simulink model "s1a"  (Simulink 2.00)
settings: Solver=ode15s  StartTime=0.0  StopTime=tstop  MaxStep=1e-3  RelTol=1e-8  AbsTol=1e-6
values from neighbouring files (symbols this model uses):
  Psi1o = 0    [M1.M]    (also in M4.M)
  Psip2o = 0    [M1.M]    (also in M4.M)
  r1 = 0.25    [M1.M]    (also in M4.M)
  rp2 = 0.134    [M1.M]    (also in M4.M)
  wb = 2*pi*Frated    (= 376.991118431)    [M1.M]    (also in M4.M)
  xl1 = 0.056    [M1.M]    (also in M4.M)
  xM = 1/(1/xm + 1/xl1 + 1/xpl2)    (= 0.0279988939489)    [M1.M]    (also in M4.M)
  xpl2 = 0.056    [M1.M]    (also in M4.M)
settings Model: SaveTime=off  SaveOutput=off  ConsistencyChecking=off

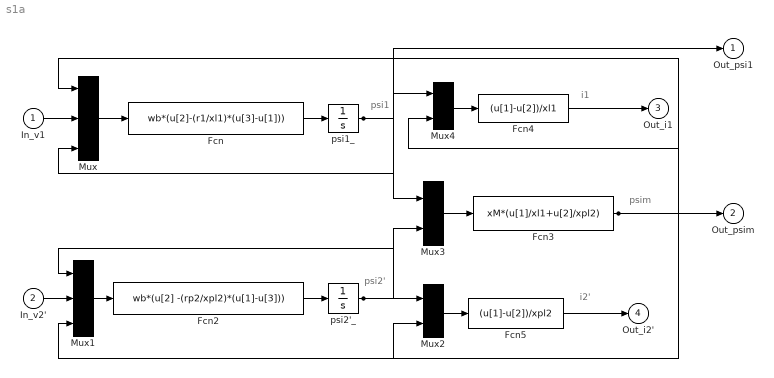
== system s1a ==
  note: i2'
  note: psi1
  note: psi2'
  note: i1
  note: psim
  In_v1 : Inport  Port=1  PortWidth=-1  SampleTime=-1
  In_v2' : Inport  Port=2  PortWidth=-1  SampleTime=-1
  Fcn : Fcn  Expr=wb*(u[2]-(r1/xl1)*(u[3]-u[1]))
  Fcn2 : Fcn  Expr=wb*(u[2] -(rp2/xpl2)*(u[1]-u[3]))
  Fcn3 : Fcn  Expr=xM*(u[1]/xl1+u[2]/xpl2)
  Fcn4 : Fcn  Expr=(u[1]-u[2])/xl1
  Fcn5 : Fcn  Expr=(u[1]-u[2])/xpl2
  Mux : Mux  Inputs=3
  Mux1 : Mux  Inputs=3
  Mux2 : Mux  Inputs=2
  Mux3 : Mux  Inputs=2
  Mux4 : Mux  Inputs=2
  psi1_ : Integrator  ExternalReset=none  InitialConditionSource=internal  InitialCondition=Psi1o  LimitOutput=off  UpperSaturationLimit=inf  LowerSaturationLimit=-inf  ShowSaturationPort=off  ShowStatePort=off  AbsoluteTolerance=auto
  psi2'_ : Integrator  ExternalReset=none  InitialConditionSource=internal  InitialCondition=Psip2o  LimitOutput=off  UpperSaturationLimit=inf  LowerSaturationLimit=-inf  ShowSaturationPort=off  ShowStatePort=off  AbsoluteTolerance=auto
  Out_psi1 : Outport  Port=1  InitialOutput=0
  Out_psim : Outport  Port=2  InitialOutput=0
  Out_i1 : Outport  Port=3  InitialOutput=0
  Out_i2' : Outport  Port=4  InitialOutput=0
  wires:
  In_v1/1 -> Mux/2
  Mux/1 -> Fcn/1
  Fcn/1 -> psi1_/1
  Fcn2/1 -> psi2'_/1
  Mux3/1 -> Fcn3/1
  Mux4/1 -> Fcn4/1
  psi1_/1 -> Mux3/1, Mux4/1, Out_psi1/1, Mux/3
  Fcn3/1 -> Mux4/2, Mux1/3, Mux/1, Out_psim/1, Mux2/2
  Fcn4/1 -> Out_i1/1
  Mux1/1 -> Fcn2/1
  In_v2'/1 -> Mux1/2
  psi2'_/1 -> Mux1/1, Mux3/2, Mux2/1
  Mux2/1 -> Fcn5/1
  Fcn5/1 -> Out_i2'/1
